simulink model "lab6_model"  (R2022b)
settings: Solver=VariableStepAuto  StartTime=0.0  StopTime=10.0  RelTol=1e-3
undefined symbols (not defined in the file or in its folder): h, licz, mian1, ym
settings Model: Creator=karol  LastModifiedBy=karol

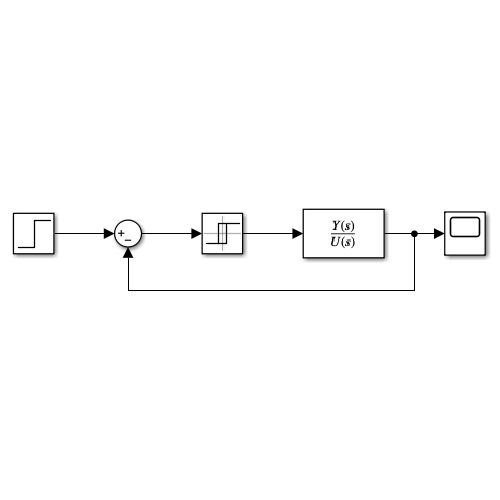
[thumbnail: Simulink's stored preview of the top-level diagram]
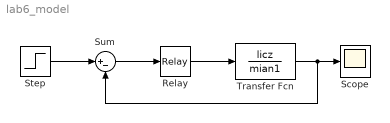
== system lab6_model ==
  Relay : Relay  OnSwitchValue=h  OffSwitchValue=-h  OnOutputValue=ym  OffOutputValue=-ym
  Scope : Scope
  Step : Step  SampleTime=0
  Sum : Sum  Inputs=|+-
  Transfer Fcn : TransferFcn  Numerator=licz  Denominator=mian1
  wires:
  Step/1 -> Sum/1
  Sum/1 -> Relay/1
  Relay/1 -> Transfer Fcn/1
  Transfer Fcn/1 -> Sum/2, Scope/1
